simulink model "ModeleFS"  (R2013a)
settings: Solver=ode3  StartTime=0.0  StopTime=T_simu  FixedStep=Pas_simu  RelTol=1e-3
values from neighbouring files (symbols this model uses):
  coeff_adh = 1.5    [Donnees_Modele_FS.m]    (also in acceleration.m = 1.55; acceleration10_12_10no.m = 1.55; acceleration12_14_10no.m = 1.55; acceleration4_6_10.m = 1.55)
  coeff_roul = 0.01    [Donnees_Modele_FS.m]    (also in acceleration.m; acceleration10_12_10no.m; acceleration12_14_10no.m; acceleration4_6_10.m)
  Couple_moteur = [0 4.6 5.2 5.4 5.2 4.9 5 5.2 5.8 6 6 5.9 5.8 5.6 5.3 4.9 4.5 4.1 3.7 3.3]    [Donnees_Modele_FS.m]
  Cx = 0.25    [Donnees_Modele_FS.m]
  D_roue = 0.53    [Donnees_Modele_FS.m]    (also in acceleration.m = 0.52; acceleration10_12_10no.m = 0.52; acceleration12_14_10no.m = 0.52; acceleration4_6_10.m = 0.52)
  Duree_chgt_rapport = 0.2    [Donnees_Modele_FS.m]
  Empatt = 1.610    (= 1.61)    [Donnees_Modele_FS.m]
  g = 9.81    [Donnees_Modele_FS.m]    (also in acceleration.m; acceleration10_12_10no.m; acceleration12_14_10no.m; acceleration4_6_10.m)
  J_eq = J_trans + J_rot    (= 22.33155)    [Donnees_Modele_FS.m]    (also in acceleration.m = 21.18; acceleration10_12_10no.m = 21.18; acceleration12_14_10no.m = 21.18; acceleration4_6_10.m = 21.18)
  Long_piste = 75    [Donnees_Modele_FS.m]
  m = m_v + m_p    (= 318)    [Donnees_Modele_FS.m]    (also in acceleration.m = 300; acceleration10_12_10no.m = 300; acceleration12_14_10no.m = 300; acceleration4_6_10.m = 300)
  Nombre_rapport = 6    [Donnees_Modele_FS.m]
  Pertes_trans = 0.95    [Donnees_Modele_FS.m]
  Rapp_engage = (1:1:6)    [Donnees_Modele_FS.m]
  Rapp_fin = 13/45    (= 0.288888888889)    [Donnees_Modele_FS.m]
  Rapp_prim = 36/76    (= 0.473684210526)    [Donnees_Modele_FS.m]
  Rapp_reduc = zeros(6,1)    [Donnees_Modele_FS.m]
  Rapport_init = 1    [Donnees_Modele_FS.m]
  Rapport_max = 4    [Donnees_Modele_FS.m]
  Regime_init = Regime_patinage    (= 9000)    [Donnees_Modele_FS.m]
  Regime_moteur = [0 4500:500:13500]    [Donnees_Modele_FS.m]
  Regime_patinage = 9000    [Donnees_Modele_FS.m]
  Regime_rupteur = 14000    [Donnees_Modele_FS.m]
  Repart_arriere = 0.53    [Donnees_Modele_FS.m]
  S = 0.4    [Donnees_Modele_FS.m]
  z_g = 0.3    [Donnees_Modele_FS.m]
undefined symbols (not defined in the file or in its folder): DiscIntNeverNeededParam
libraries: simulink x1
settings Model: Creator=Sebastien  LastModifiedBy=Sebastien

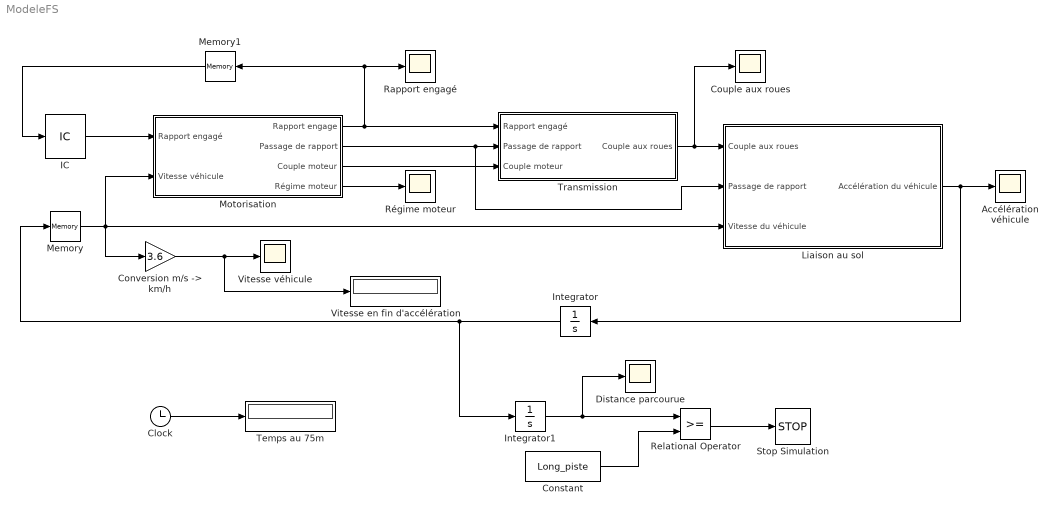
== system ModeleFS ==
  Accélération véhicule : Scope
  Clock : Clock
  Constant : Constant  Value=Long_piste
  "Conversion m/s -> km/h" : Gain  Gain=3.6
  Couple aux roues : Scope
      settings: TimeRange=20  SaveName=ScopeData3
  Distance parcourue : Scope
      settings: TimeRange=20  SaveName=ScopeData11
  IC : InitialCondition  Value=Rapport_init
  Integrator : Integrator
  Integrator1 : Integrator
  Liaison au sol : Subsystem
  Memory : Memory
  Memory1 : Memory
  Motorisation : Subsystem
  Rapport engagé : Scope
      settings: SaveName=ScopeData6
  Relational Operator : RelationalOperator  OutDataTypeStr=boolean
  Régime moteur : Scope
      settings: TimeRange=20  SaveName=ScopeData9
  Stop Simulation : Stop
  Temps au 75m : Display
  Transmission : Subsystem
  Vitesse en fin d'accélération : Display
  Vitesse véhicule : Scope
      settings: TimeRange=20  SaveName=ScopeData2
  wires:
  Motorisation/3(Couple moteur) -> Transmission/3(Couple moteur)
  Transmission/1(Couple aux roues) -> Couple aux roues/1, Liaison au sol/1(Couple aux roues)
  Liaison au sol/1(Accélération du véhicule) -> Accélération véhicule/1, Integrator/1
  Memory/1 -> "Conversion m/s -> km/h"/1, Liaison au sol/3(Vitesse du véhicule), Motorisation/2(Vitesse véhicule)
  Integrator/1 -> Integrator1/1, Memory/1
  Motorisation/2(Passage de rapport) -> Liaison au sol/2(Passage de rapport), Transmission/2(Passage de rapport)
  IC/1 -> Motorisation/1(Rapport engagé)
  Motorisation/4(Régime moteur) -> Régime moteur/1
  Integrator1/1 -> Distance parcourue/1, Relational Operator/1
  "Conversion m/s -> km/h"/1 -> Vitesse en fin d'accélération/1, Vitesse véhicule/1
  Constant/1 -> Relational Operator/2
  Relational Operator/1 -> Stop Simulation/1
  Clock/1 -> Temps au 75m/1
  Motorisation/1(Rapport engage) -> Transmission/1(Rapport engagé), Rapport engagé/1, Memory1/1
  Memory1/1 -> IC/1

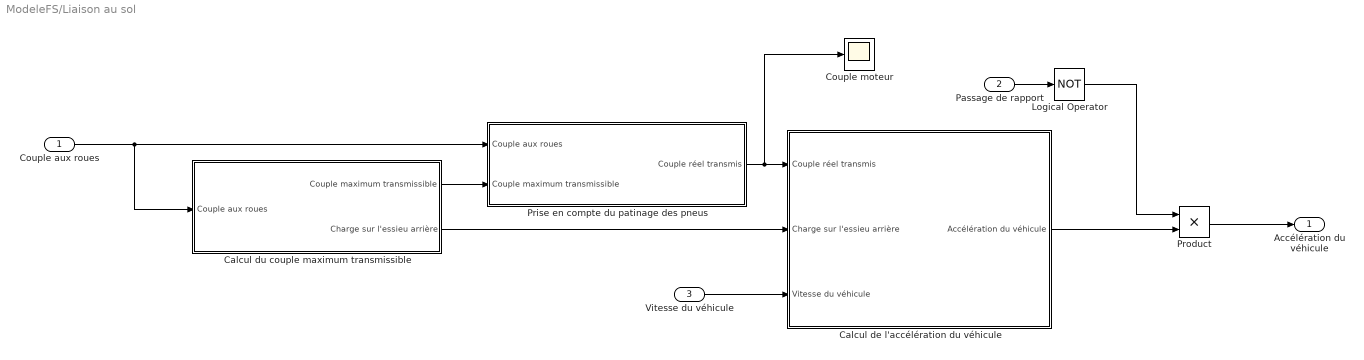
== system ModeleFS/Liaison au sol ==
  Couple aux roues : Inport
  Passage de rapport : Inport  Port=2
  Vitesse du véhicule : Inport  Port=3
  Calcul de l'accélération du véhicule : Subsystem
  Calcul du couple maximum transmissible : Subsystem
  Couple moteur : Scope
      settings: TimeRange=20
  Logical Operator : Logic  Operator=NOT  AllPortsSameDT=off  OutDataTypeStr=boolean
  Prise en compte du patinage des pneus : Subsystem
  Product : Product
  Accélération du véhicule : Outport
  wires:
  Couple aux roues/1 -> Calcul du couple maximum transmissible/1(Couple aux roues), Prise en compte du patinage des pneus/1(Couple aux roues)
  Prise en compte du patinage des pneus/1(Couple réel transmis) -> Couple moteur/1, Calcul de l'accélération du véhicule/1(Couple réel transmis)
  Calcul du couple maximum transmissible/2(Charge sur l'essieu arrière) -> Calcul de l'accélération du véhicule/2(Charge sur l'essieu arrière)
  Passage de rapport/1 -> Logical Operator/1
  Calcul de l'accélération du véhicule/1(Accélération du véhicule) -> Product/2
  Logical Operator/1 -> Product/1
  Product/1 -> Accélération du véhicule/1
  Vitesse du véhicule/1 -> Calcul de l'accélération du véhicule/3(Vitesse du véhicule)
  Calcul du couple maximum transmissible/1(Couple maximum transmissible) -> Prise en compte du patinage des pneus/2(Couple maximum transmissible)

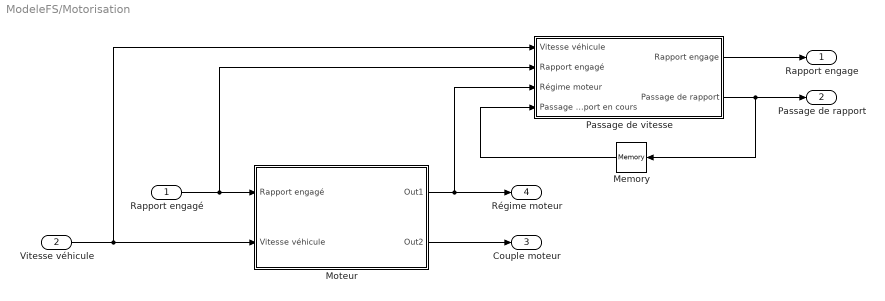
== system ModeleFS/Motorisation ==
  Rapport engagé : Inport
  Vitesse véhicule : Inport  Port=2
  Memory : Memory
  Moteur : Subsystem
  Passage de vitesse : Subsystem
  Rapport engage : Outport
  Passage de rapport : Outport  Port=2
  Couple moteur : Outport  Port=3
  Régime moteur : Outport  Port=4
  wires:
  Rapport engagé/1 -> Passage de vitesse/2(Rapport engagé), Moteur/1(Rapport engagé)
  Moteur/1(Out1) -> Passage de vitesse/3(Régime moteur), Régime moteur/1
  Moteur/2(Out2) -> Couple moteur/1
  Passage de vitesse/2(Passage de rapport) -> Memory/1, Passage de rapport/1
  Vitesse véhicule/1 -> Passage de vitesse/1(Vitesse véhicule), Moteur/2(Vitesse véhicule)
  Passage de vitesse/1(Rapport engage) -> Rapport engage/1
  Memory/1 -> Passage de vitesse/4(Passage de rapport en cours)

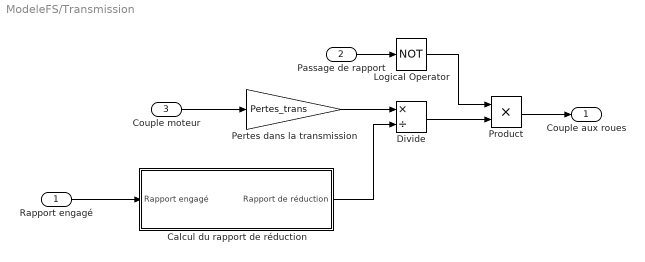
== system ModeleFS/Transmission ==
  Rapport engagé : Inport
  Passage de rapport : Inport  Port=2
  Couple moteur : Inport  Port=3
  Calcul du rapport de réduction : Subsystem
  Divide : Product  Inputs=*/
  Logical Operator : Logic  Operator=NOT  AllPortsSameDT=off  OutDataTypeStr=boolean
  Pertes dans la transmission : Gain  Gain=Pertes_trans
  Product : Product
  Couple aux roues : Outport
  wires:
  Rapport engagé/1 -> Calcul du rapport de réduction/1(Rapport engagé)
  Couple moteur/1 -> Pertes dans la transmission/1
  Pertes dans la transmission/1 -> Divide/1
  Calcul du rapport de réduction/1(Rapport de réduction) -> Divide/2
  Passage de rapport/1 -> Logical Operator/1
  Divide/1 -> Product/2
  Logical Operator/1 -> Product/1
  Product/1 -> Couple aux roues/1

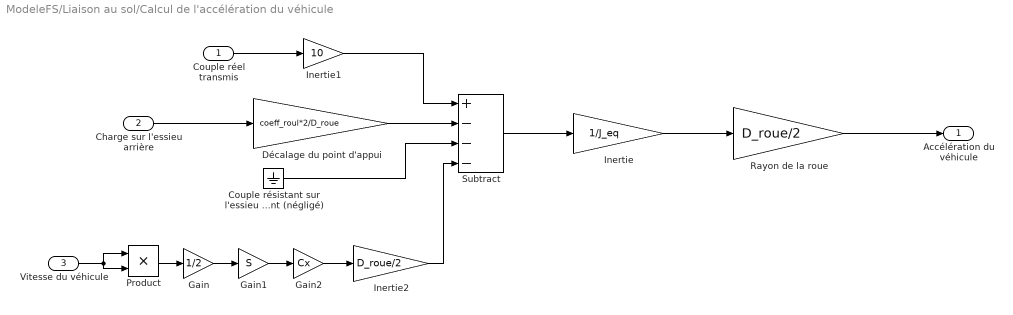
== system ModeleFS/Liaison au sol/Calcul de l'accélération du véhicule ==
  Couple réel transmis : Inport
  Charge sur l'essieu arrière : Inport  Port=2
  Vitesse du véhicule : Inport  Port=3
  Couple résistant sur l'essieu avant (négligé) : Ground
  Décalage du point d'appui : Gain  Gain=coeff_roul*2/D_roue
  Gain : Gain  Gain=1/2
  Gain1 : Gain  Gain=S
  Gain2 : Gain  Gain=Cx
  Inertie : Gain  Gain=1/J_eq
  Inertie1 : Gain  Gain=10
  Inertie2 : Gain  Gain=D_roue/2
  Product : Product
  Rayon de la roue : Gain  Gain=D_roue/2
  Subtract : Sum  Inputs=+---
  Accélération du véhicule : Outport
  wires:
  Subtract/1 -> Inertie/1
  Inertie/1 -> Rayon de la roue/1
  Charge sur l'essieu arrière/1 -> Décalage du point d'appui/1
  Couple réel transmis/1 -> Inertie1/1
  Inertie1/1 -> Subtract/1
  Décalage du point d'appui/1 -> Subtract/2
  Couple résistant sur l'essieu avant (négligé)/1 -> Subtract/3
  Gain/1 -> Gain1/1
  Gain1/1 -> Gain2/1
  Product/1 -> Gain/1
  Vitesse du véhicule/1 -> Product/1, Product/2
  Gain2/1 -> Inertie2/1
  Inertie2/1 -> Subtract/4
  Rayon de la roue/1 -> Accélération du véhicule/1

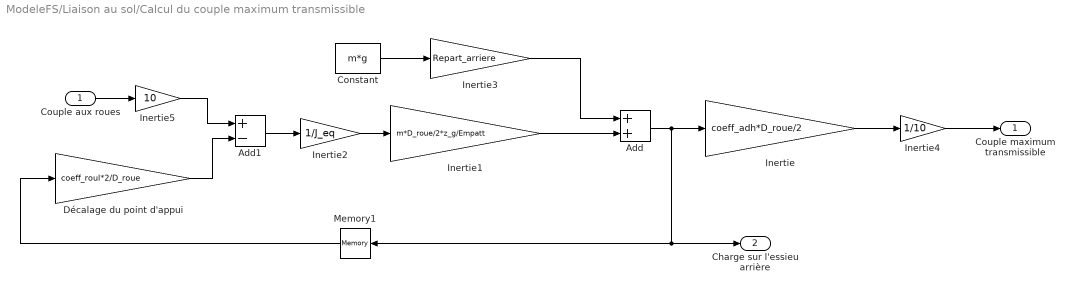
== system ModeleFS/Liaison au sol/Calcul du couple maximum transmissible ==
  Couple aux roues : Inport
  Add : Sum
  Add1 : Sum  Inputs=+-
  Constant : Constant  Value=m*g
  Décalage du point d'appui : Gain  Gain=coeff_roul*2/D_roue
  Inertie : Gain  Gain=coeff_adh*D_roue/2
  Inertie1 : Gain  Gain=m*D_roue/2*z_g/Empatt
  Inertie2 : Gain  Gain=1/J_eq
  Inertie3 : Gain  Gain=Repart_arriere
  Inertie4 : Gain  Gain=1/10
  Inertie5 : Gain  Gain=10
  Memory1 : Memory
  Couple maximum transmissible : Outport
  Charge sur l'essieu arrière : Outport  Port=2
  wires:
  Inertie1/1 -> Add/2
  Add/1 -> Memory1/1, Charge sur l'essieu arrière/1, Inertie/1
  Inertie3/1 -> Add/1
  Couple aux roues/1 -> Inertie5/1
  Constant/1 -> Inertie3/1
  Inertie4/1 -> Couple maximum transmissible/1
  Inertie/1 -> Inertie4/1
  Inertie2/1 -> Inertie1/1
  Add1/1 -> Inertie2/1
  Inertie5/1 -> Add1/1
  Décalage du point d'appui/1 -> Add1/2
  Memory1/1 -> Décalage du point d'appui/1

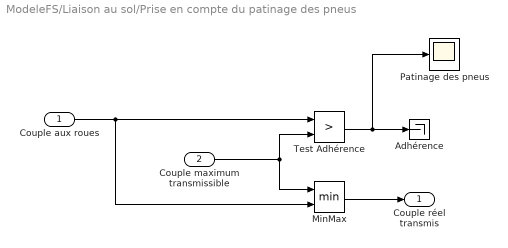
== system ModeleFS/Liaison au sol/Prise en compte du patinage des pneus ==
  Couple aux roues : Inport
  Couple maximum transmissible : Inport  Port=2
  Adhérence : Terminator
  MinMax : MinMax  Inputs=2
  Patinage des pneus : Scope
      settings: TimeRange=20  SaveName=ScopeData4
  Test Adhérence : RelationalOperator  Operator=>  OutDataTypeStr=boolean
  Couple réel transmis : Outport
  wires:
  Test Adhérence/1 -> Patinage des pneus/1, Adhérence/1
  MinMax/1 -> Couple réel transmis/1
  Couple maximum transmissible/1 -> MinMax/1, Test Adhérence/2
  Couple aux roues/1 -> MinMax/2, Test Adhérence/1

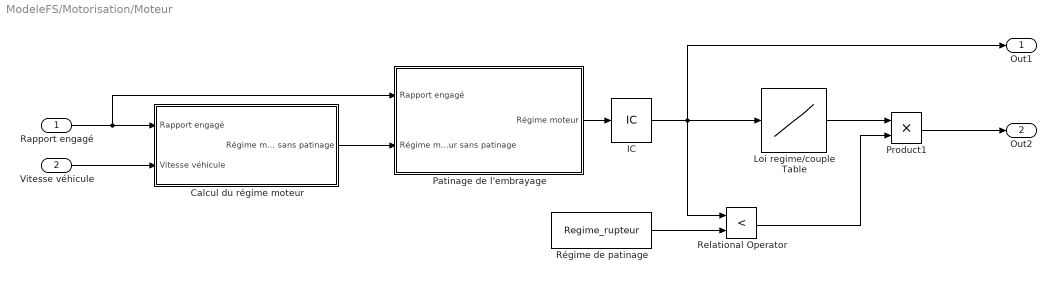
== system ModeleFS/Motorisation/Moteur ==
  Rapport engagé : Inport
  Vitesse véhicule : Inport  Port=2
  Calcul du régime moteur : Subsystem
  IC : InitialCondition  Value=Regime_init
  Loi regime/couple Table : Lookup_n-D  NumberOfTableDimensions=1  BreakpointsForDimension1=Regime_moteur  Table=Couple_moteur  RndMeth=Simplest  InputSameDT=on
  Patinage de l'embrayage : Subsystem
  Product1 : Product
  Relational Operator : RelationalOperator  Operator=<  OutDataTypeStr=boolean
  Régime de patinage : Constant  Value=Regime_rupteur
  Out1 : Outport
  Out2 : Outport  Port=2
  wires:
  Patinage de l'embrayage/1(Régime moteur) -> IC/1
  Calcul du régime moteur/1(Régime moteur sans patinage) -> Patinage de l'embrayage/2(Régime moteur sans patinage)
  Relational Operator/1 -> Product1/2
  Product1/1 -> Out2/1
  Régime de patinage/1 -> Relational Operator/2
  IC/1 -> Out1/1, Loi regime/couple Table/1, Relational Operator/1
  Vitesse véhicule/1 -> Calcul du régime moteur/2(Vitesse véhicule)
  Rapport engagé/1 -> Patinage de l'embrayage/1(Rapport engagé), Calcul du régime moteur/1(Rapport engagé)
  Loi regime/couple Table/1 -> Product1/1

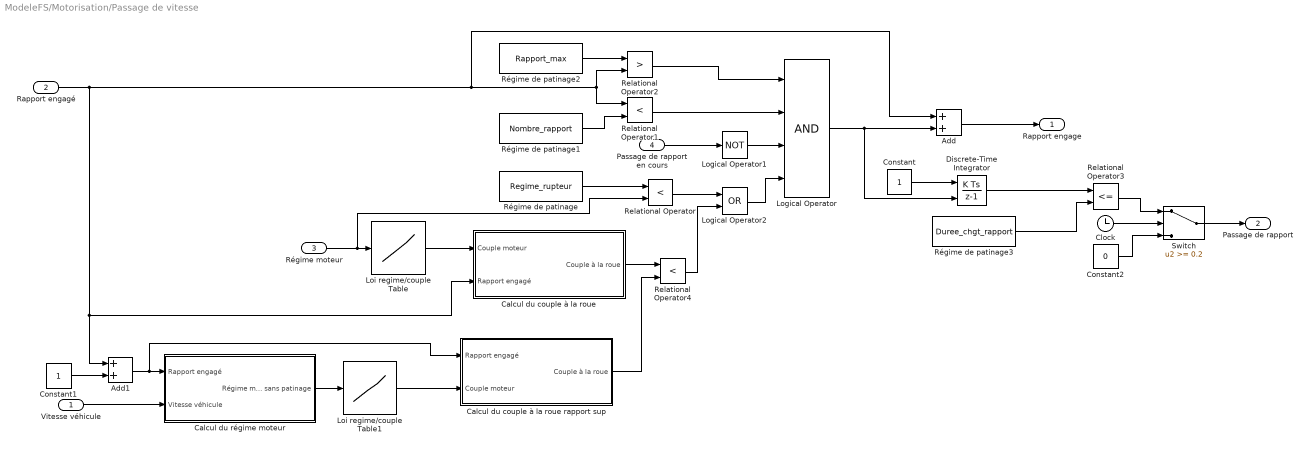
== system ModeleFS/Motorisation/Passage de vitesse ==
  Vitesse véhicule : Inport
  Rapport engagé : Inport  Port=2
  Régime moteur : Inport  Port=3
  Passage de rapport en cours : Inport  Port=4
  Add : Sum
  Add1 : Sum
  Calcul du couple à la roue : Subsystem
  Calcul du couple à la roue rapport sup : Subsystem
  Calcul du régime moteur : Subsystem
  Clock : Clock
  Constant : Constant
  Constant1 : Constant
  Constant2 : Constant  Value=0
  Discrete-Time Integrator : DiscreteIntegrator  ExternalReset=rising  SampleTime=-1  ICPrevOutput=DiscIntNeverNeededParam  ICPrevScaledInput=DiscIntNeverNeededParam
  Logical Operator : Logic  Inputs=4  AllPortsSameDT=off  OutDataTypeStr=boolean
  Logical Operator1 : Logic  Operator=NOT  AllPortsSameDT=off  OutDataTypeStr=boolean
  Logical Operator2 : Logic  Operator=OR  AllPortsSameDT=off  OutDataTypeStr=boolean
  Loi regime/couple Table : Lookup_n-D  NumberOfTableDimensions=1  BreakpointsForDimension1=Regime_moteur  Table=Couple_moteur  RndMeth=Simplest  InputSameDT=on
  Loi regime/couple Table1 : Lookup_n-D  NumberOfTableDimensions=1  BreakpointsForDimension1=Regime_moteur  Table=Couple_moteur  RndMeth=Simplest  InputSameDT=on
  Relational Operator : RelationalOperator  Operator=<  OutDataTypeStr=boolean
  Relational Operator1 : RelationalOperator  Operator=<  OutDataTypeStr=boolean
  Relational Operator2 : RelationalOperator  Operator=>  OutDataTypeStr=boolean
  Relational Operator3 : RelationalOperator  Operator=<=  OutDataTypeStr=boolean
  Relational Operator4 : RelationalOperator  Operator=<  OutDataTypeStr=boolean
  Régime de patinage : Constant  Value=Regime_rupteur
  Régime de patinage1 : Constant  Value=Nombre_rapport
  Régime de patinage2 : Constant  Value=Rapport_max
  Régime de patinage3 : Constant  Value=Duree_chgt_rapport
  Switch : Switch  Threshold=0.2
  Rapport engage : Outport
  Passage de rapport : Outport  Port=2
  wires:
  Régime de patinage/1 -> Relational Operator/1
  Régime moteur/1 -> Relational Operator/2, Loi regime/couple Table/1
  Rapport engagé/1 -> Add/1, Relational Operator2/2, Relational Operator1/1, Calcul du couple à la roue/2(Rapport engagé), Add1/1
  Relational Operator1/1 -> Logical Operator/2
  Relational Operator2/1 -> Logical Operator/1
  Relational Operator/1 -> Logical Operator2/1
  Régime de patinage1/1 -> Relational Operator1/2
  Régime de patinage2/1 -> Relational Operator2/1
  Add/1 -> Rapport engage/1
  Logical Operator/1 -> Discrete-Time Integrator/2, Add/2
  Discrete-Time Integrator/1 -> Relational Operator3/1
  Relational Operator3/1 -> Switch/1
  Régime de patinage3/1 -> Relational Operator3/2
  Logical Operator1/1 -> Logical Operator/3
  Passage de rapport en cours/1 -> Logical Operator1/1
  Constant/1 -> Discrete-Time Integrator/1
  Vitesse véhicule/1 -> Calcul du régime moteur/2(Vitesse véhicule)
  Add1/1 -> Calcul du couple à la roue rapport sup/1(Rapport engagé), Calcul du régime moteur/1(Rapport engagé)
  Constant1/1 -> Add1/2
  Calcul du régime moteur/1(Régime moteur sans patinage) -> Loi regime/couple Table1/1
  Loi regime/couple Table1/1 -> Calcul du couple à la roue rapport sup/2(Couple moteur)
  Loi regime/couple Table/1 -> Calcul du couple à la roue/1(Couple moteur)
  Relational Operator4/1 -> Logical Operator2/2
  Logical Operator2/1 -> Logical Operator/4
  Calcul du couple à la roue/1(Couple à la roue) -> Relational Operator4/1
  Calcul du couple à la roue rapport sup/1(Couple à la roue) -> Relational Operator4/2
  Switch/1 -> Passage de rapport/1
  Constant2/1 -> Switch/3
  Clock/1 -> Switch/2

== system ModeleFS/Transmission/Calcul du rapport de réduction ==
  Rapport engagé : Inport
  Rapport de reduction BV Table : Lookup_n-D  NumberOfTableDimensions=1  BreakpointsForDimension1=Rapp_engage  Table=Rapp_reduc  RndMeth=Simplest  InputSameDT=on
  Rapport final : Gain  Gain=Rapp_fin
  Rapport primaire : Gain  Gain=Rapp_prim
  Rapport de réduction : Outport
  wires:
  Rapport final/1 -> Rapport de réduction/1
  Rapport engagé/1 -> Rapport de reduction BV Table/1
  Rapport primaire/1 -> Rapport final/1
  Rapport de reduction BV Table/1 -> Rapport primaire/1

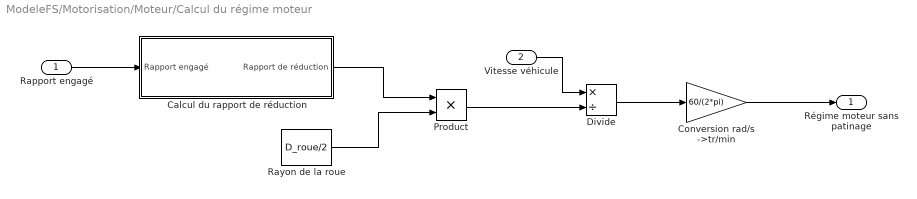
== system ModeleFS/Motorisation/Moteur/Calcul du régime moteur ==
  Rapport engagé : Inport
  Vitesse véhicule : Inport  Port=2
  Calcul du rapport de réduction : Subsystem
  Conversion rad/s ->tr/min : Gain  Gain=60/(2*pi)
  Divide : Product  Inputs=*/
  Product : Product
  Rayon de la roue : Constant  Value=D_roue/2
  Régime moteur sans patinage : Outport
  wires:
  Rapport engagé/1 -> Calcul du rapport de réduction/1(Rapport engagé)
  Vitesse véhicule/1 -> Divide/1
  Calcul du rapport de réduction/1(Rapport de réduction) -> Product/1
  Rayon de la roue/1 -> Product/2
  Product/1 -> Divide/2
  Divide/1 -> Conversion rad/s ->tr/min/1
  Conversion rad/s ->tr/min/1 -> Régime moteur sans patinage/1

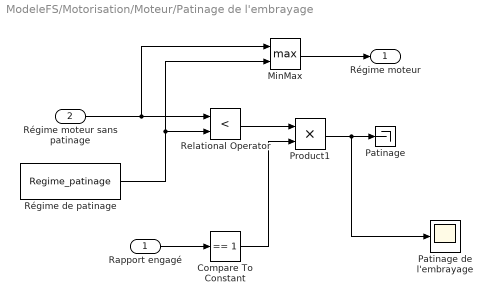
== system ModeleFS/Motorisation/Moteur/Patinage de l'embrayage ==
  Rapport engagé : Inport
  Régime moteur sans patinage : Inport  Port=2
  Compare To Constant : simulink/Logic and Bit Operations/Compare To Constant  relop===  const=1  OutDataTypeStr=boolean
  MinMax : MinMax  Function=max  Inputs=2
  Patinage : Terminator
  Patinage de l'embrayage : Scope
      settings: SaveName=ScopeData5
  Product1 : Product
  Relational Operator : RelationalOperator  Operator=<  OutDataTypeStr=boolean
  Régime de patinage : Constant  Value=Regime_patinage
  Régime moteur : Outport
  wires:
  Rapport engagé/1 -> Compare To Constant/1
  Régime moteur sans patinage/1 -> MinMax/1, Relational Operator/1
  Régime de patinage/1 -> MinMax/2, Relational Operator/2
  Relational Operator/1 -> Product1/1
  Product1/1 -> Patinage de l'embrayage/1, Patinage/1
  Compare To Constant/1 -> Product1/2
  MinMax/1 -> Régime moteur/1

== system ModeleFS/Motorisation/Passage de vitesse/Calcul du couple à la roue ==
  Couple moteur : Inport
  Rapport engagé : Inport  Port=2
  Calcul du rapport de réduction : Subsystem
  Divide : Product  Inputs=*/
  Pertes dans la transmission : Gain  Gain=Pertes_trans
  Couple à la roue : Outport
  wires:
  Rapport engagé/1 -> Calcul du rapport de réduction/1(Rapport engagé)
  Divide/1 -> Couple à la roue/1
  Couple moteur/1 -> Pertes dans la transmission/1
  Pertes dans la transmission/1 -> Divide/1
  Calcul du rapport de réduction/1(Rapport de réduction) -> Divide/2

== system ModeleFS/Motorisation/Passage de vitesse/Calcul du couple à la roue rapport sup ==
  Rapport engagé : Inport
  Couple moteur : Inport  Port=2
  Calcul du rapport de réduction : Subsystem
  Divide : Product  Inputs=*/
  Pertes dans la transmission : Gain  Gain=Pertes_trans
  Couple à la roue : Outport
  wires:
  Rapport engagé/1 -> Calcul du rapport de réduction/1(Rapport engagé)
  Divide/1 -> Couple à la roue/1
  Couple moteur/1 -> Pertes dans la transmission/1
  Pertes dans la transmission/1 -> Divide/1
  Calcul du rapport de réduction/1(Rapport de réduction) -> Divide/2

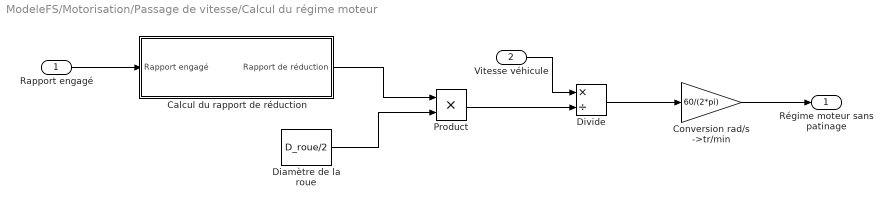
== system ModeleFS/Motorisation/Passage de vitesse/Calcul du régime moteur ==
  Rapport engagé : Inport
  Vitesse véhicule : Inport  Port=2
  Calcul du rapport de réduction : Subsystem
  Conversion rad/s ->tr/min : Gain  Gain=60/(2*pi)
  Diamètre de la roue : Constant  Value=D_roue/2
  Divide : Product  Inputs=*/
  Product : Product
  Régime moteur sans patinage : Outport
  wires:
  Rapport engagé/1 -> Calcul du rapport de réduction/1(Rapport engagé)
  Vitesse véhicule/1 -> Divide/1
  Calcul du rapport de réduction/1(Rapport de réduction) -> Product/1
  Diamètre de la roue/1 -> Product/2
  Product/1 -> Divide/2
  Divide/1 -> Conversion rad/s ->tr/min/1
  Conversion rad/s ->tr/min/1 -> Régime moteur sans patinage/1

== system ModeleFS/Motorisation/Moteur/Calcul du régime moteur/Calcul du rapport de réduction ==
  Rapport engagé : Inport
  Rapport de reduction BV Table : Lookup_n-D  NumberOfTableDimensions=1  BreakpointsForDimension1=Rapp_engage  Table=Rapp_reduc  RndMeth=Simplest  InputSameDT=on
  Rapport final : Gain  Gain=Rapp_fin
  Rapport primaire : Gain  Gain=Rapp_prim
  Rapport de réduction : Outport
  wires:
  Rapport final/1 -> Rapport de réduction/1
  Rapport engagé/1 -> Rapport de reduction BV Table/1
  Rapport primaire/1 -> Rapport final/1
  Rapport de reduction BV Table/1 -> Rapport primaire/1

== system ModeleFS/Motorisation/Passage de vitesse/Calcul du couple à la roue/Calcul du rapport de réduction ==
  Rapport engagé : Inport
  Rapport de reduction BV Table : Lookup_n-D  NumberOfTableDimensions=1  BreakpointsForDimension1=Rapp_engage  Table=Rapp_reduc  RndMeth=Simplest  InputSameDT=on
  Rapport final : Gain  Gain=Rapp_fin
  Rapport primaire : Gain  Gain=Rapp_prim
  Rapport de réduction : Outport
  wires:
  Rapport final/1 -> Rapport de réduction/1
  Rapport engagé/1 -> Rapport de reduction BV Table/1
  Rapport primaire/1 -> Rapport final/1
  Rapport de reduction BV Table/1 -> Rapport primaire/1

== system ModeleFS/Motorisation/Passage de vitesse/Calcul du couple à la roue rapport sup/Calcul du rapport de réduction ==
  Rapport engagé : Inport
  Rapport de reduction BV Table : Lookup_n-D  NumberOfTableDimensions=1  BreakpointsForDimension1=Rapp_engage  Table=Rapp_reduc  RndMeth=Simplest  InputSameDT=on
  Rapport final : Gain  Gain=Rapp_fin
  Rapport primaire : Gain  Gain=Rapp_prim
  Rapport de réduction : Outport
  wires:
  Rapport final/1 -> Rapport de réduction/1
  Rapport engagé/1 -> Rapport de reduction BV Table/1
  Rapport primaire/1 -> Rapport final/1
  Rapport de reduction BV Table/1 -> Rapport primaire/1

== system ModeleFS/Motorisation/Passage de vitesse/Calcul du régime moteur/Calcul du rapport de réduction ==
  Rapport engagé : Inport
  Rapport de reduction BV Table : Lookup_n-D  NumberOfTableDimensions=1  BreakpointsForDimension1=Rapp_engage  Table=Rapp_reduc  RndMeth=Simplest  InputSameDT=on
  Rapport final : Gain  Gain=Rapp_fin
  Rapport primaire : Gain  Gain=Rapp_prim
  Rapport de réduction : Outport
  wires:
  Rapport final/1 -> Rapport de réduction/1
  Rapport engagé/1 -> Rapport de reduction BV Table/1
  Rapport primaire/1 -> Rapport final/1
  Rapport de reduction BV Table/1 -> Rapport primaire/1
